simulink model "comprig_mpc"  (Simulink 8.6)
settings: Solver=ode15s  StartTime=0.0  StopTime=300  RelTol=1e-5
InitFcn:
  | MpcSetup
StartFcn:
  | MpcSetup
values from neighbouring files (symbols this model uses):
  x_init_lin = [0.898 ... (first row only)    [MpcSetup.m]    (also in MpcSetup_linearized.m; compressor_setup.m; setup_compressor.m; test2.m = [0.899; 1.125; 0.1512; 440.7; 0])
settings Model: Creator=chmemer  LastModifiedBy=chkajon
settings DebuggingCC: FcnCallInpInsideContextMsg=UseLocalSettings

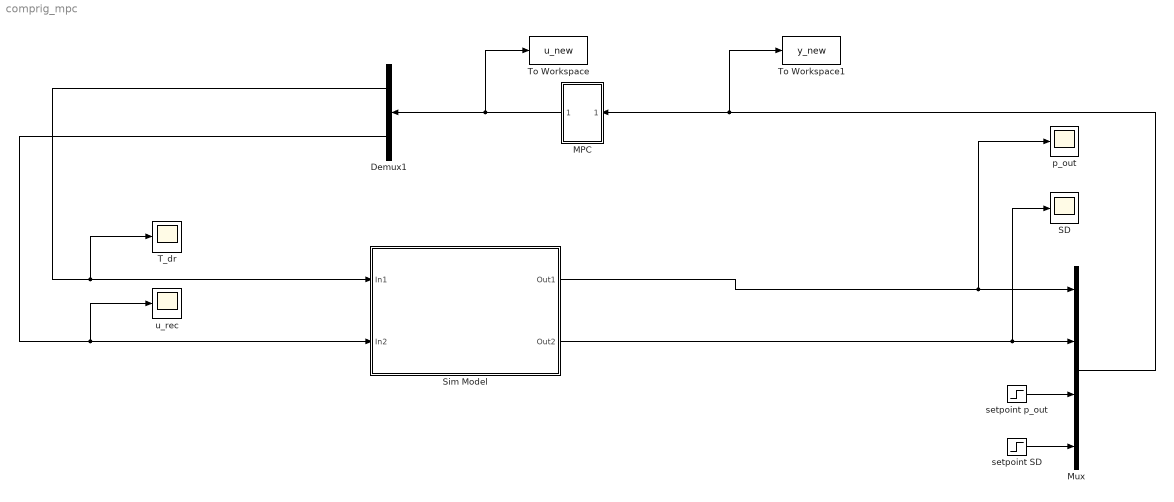
== system comprig_mpc ==
  Demux1 : Demux  Outputs=2
  MPC : Subsystem
  Mux : Mux
  SD : Scope
  Sim Model : Subsystem
  T_dr : Scope
  To Workspace : ToWorkspace  VariableName=u_new  SaveFormat=Timeseries  SampleTime=-1
  To Workspace1 : ToWorkspace  VariableName=y_new  SaveFormat=Timeseries  SampleTime=-1
  p_out : Scope
  setpoint SD : Step  After=0  SampleTime=0
  setpoint p_out : Step  After=0  SampleTime=0
  u_rec : Scope
  wires:
  Demux1/1 -> T_dr/1, Sim Model/1(In1)
  setpoint p_out/1 -> Mux/3
  setpoint SD/1 -> Mux/4
  Demux1/2 -> u_rec/1, Sim Model/2(In2)
  Mux/1 -> To Workspace1/1, MPC/1(In1)
  MPC/1(Out1) -> To Workspace/1, Demux1/1
  Sim Model/1(Out1) -> Mux/1, p_out/1
  Sim Model/2(Out2) -> Mux/2, SD/1

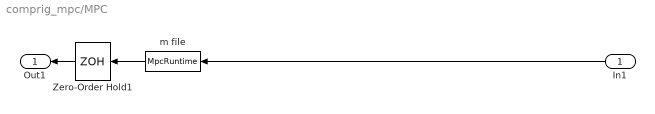
== system comprig_mpc/MPC ==
  In1 : Inport
  Zero-Order Hold1 : ZeroOrderHold  SampleTime=0.05
  m file : S-Function  FunctionName=MpcRuntime  Parameters=[],[]  SFunctionDeploymentMode=off  EnableBusSupport=off
  Out1 : Outport
  wires:
  m file/1 -> Zero-Order Hold1/1
  In1/1 -> m file/1
  Zero-Order Hold1/1 -> Out1/1

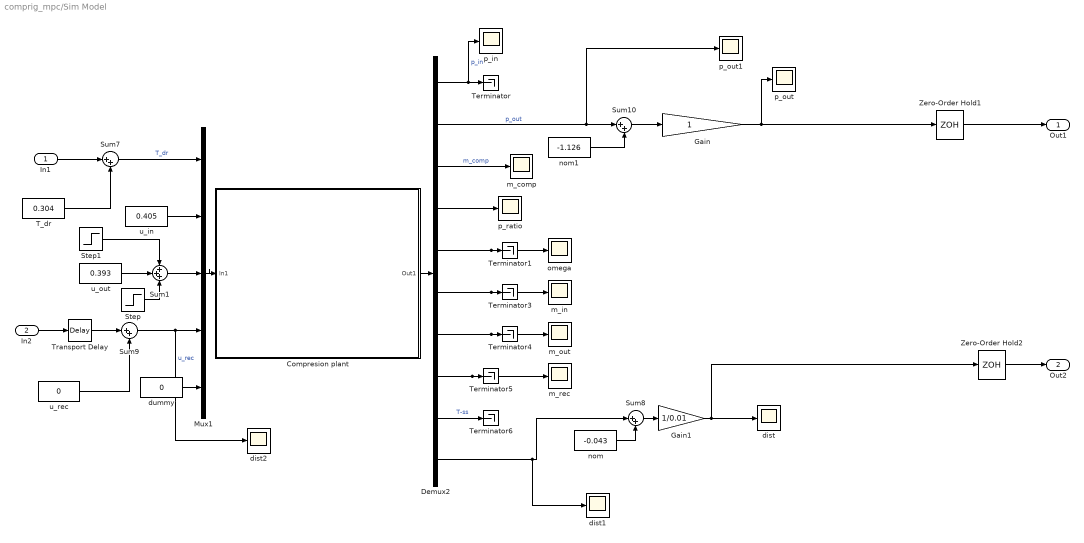
== system comprig_mpc/Sim Model ==
  In1 : Inport
  In2 : Inport  Port=2
  Compresion plant : Subsystem
      mask Display: image(imread('comp_plant.jpg'))
  Demux2 : Demux  Outputs=10
  Gain : Gain
  Gain1 : Gain  Gain=1/0.01
  Mux1 : Mux  Inputs=5
  Step : Step  Time=50  After=0  SampleTime=0
  Step1 : Step  Time=100  After=-0.1  SampleTime=0
  Sum1 : Sum  Inputs=+++
  Sum{7..10} (4 alike) : Sum  Inputs=|++
  T_dr : Constant  Value=0.304
  Terminator{,1,3..6} (6 alike) : Terminator
  Transport Delay : TransportDelay  DelayTime=1.0
  Zero-Order Hold1 : ZeroOrderHold  SampleTime=0.05
  Zero-Order Hold2 : ZeroOrderHold  SampleTime=0.05
  dist : Scope
  dist1 : Scope
  dist2 : Scope
  dummy : Constant  Value=0
  m_comp : Scope
  m_in : Scope
  m_out : Scope
  m_rec : Scope
  nom : Constant  Value=-0.043
  nom1 : Constant  Value=-1.126
  omega : Scope
  p_in : Scope
  p_out : Scope
  p_out1 : Scope
  p_ratio : Scope
  u_in : Constant  Value=0.405
  u_out : Constant  Value=0.393
  u_rec : Constant  Value=0
  Out1 : Outport
  Out2 : Outport  Port=2
  wires:
  Compresion plant/1(Out1) -> Demux2/1
  Mux1/1 -> Compresion plant/1(In1)
  Demux2/3 -> m_comp/1  "m_comp"
  u_in/1 -> Mux1/2
  Demux2/6 -> Terminator3/1, m_in/1
  Demux2/8 -> Terminator5/1, m_rec/1
  Demux2/7 -> Terminator4/1, m_out/1
  In2/1 -> Transport Delay/1
  Sum7/1 -> Mux1/1  "T_dr"
  Sum9/1 -> Mux1/4, dist2/1  "u_rec"
  nom/1 -> Sum8/2
  Sum8/1 -> Gain1/1
  Demux2/2 -> Sum10/1, p_out1/1  "p_out"
  Demux2/1 -> Terminator/1, p_in/1  "p_in"
  Demux2/5 -> Terminator1/1, omega/1
  Demux2/4 -> p_ratio/1
  Sum10/1 -> Gain/1
  nom1/1 -> Sum10/2
  Gain/1 -> p_out/1, Zero-Order Hold1/1
  T_dr/1 -> Sum7/2
  u_rec/1 -> Sum9/2
  In1/1 -> Sum7/1
  Gain1/1 -> dist/1, Zero-Order Hold2/1
  Demux2/10 -> Sum8/1, dist1/1
  dummy/1 -> Mux1/5
  Zero-Order Hold2/1 -> Out2/1
  Zero-Order Hold1/1 -> Out1/1
  Transport Delay/1 -> Sum9/1
  Sum1/1 -> Mux1/3
  Demux2/9 -> Terminator6/1  "T-ss"
  u_out/1 -> Sum1/2
  Step/1 -> Sum1/3
  Step1/1 -> Sum1/1

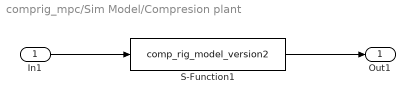
== system comprig_mpc/Sim Model/Compresion plant ==
  In1 : Inport
  S-Function1 : S-Function  FunctionName=comp_rig_model_version2  Parameters=[], x_init_lin  SFunctionDeploymentMode=off  EnableBusSupport=off
  Out1 : Outport
  wires:
  S-Function1/1 -> Out1/1
  In1/1 -> S-Function1/1
